simulink model "qnetdcmotor_AhmedMohsin"  (R2022a)
settings: Solver=VariableStepAuto  StartTime=0.0  StopTime=10.0  RelTol=1e-3
InitFcn:
  | R=8.70
  | kt=0.0334
  | ke=0.0334
  | J=1.80e-6
  | L=0.00
  | b=0.00
settings Model: Creator=ahmed  LastModifiedBy=ahmed

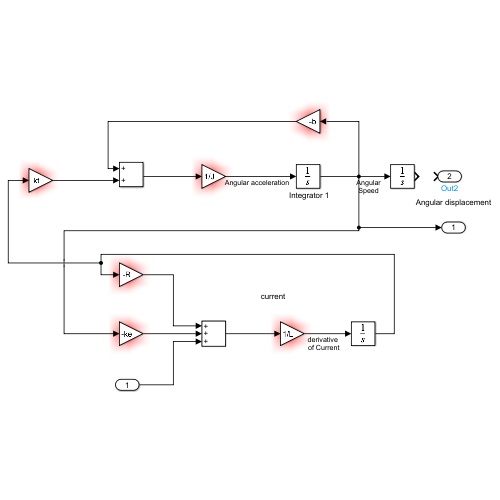
[thumbnail: Simulink's stored preview of the top-level diagram]
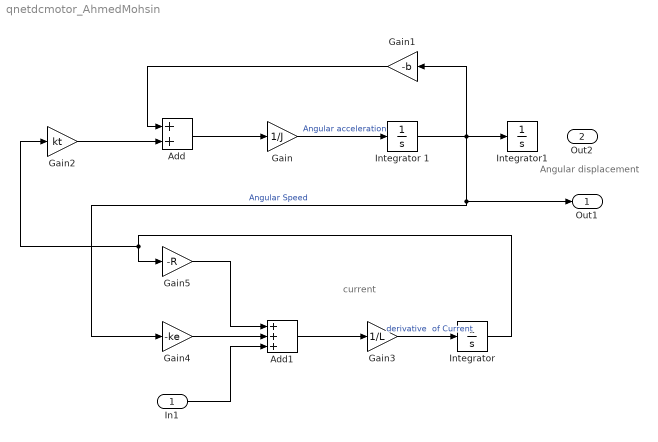
== system qnetdcmotor_AhmedMohsin ==
  note: current
  note: Angular displacement
  In1 : Inport
  " Integrator 1" : Integrator
  Add : Sum
  Add1 : Sum  Inputs=+++
  Gain : Gain  Gain=1/J
  Gain1 : Gain  Gain=-b
  Gain2 : Gain  Gain=kt
  Gain3 : Gain  Gain=1/L
  Gain4 : Gain  Gain=-ke
  Gain5 : Gain  Gain=-R
  Integrator : Integrator
  Integrator1 : Integrator
  Out1 : Outport
  Out2 : Outport  Port=2
  wires:
  " Integrator 1"/1 -> Gain4/1, Out1/1, Gain1/1, Integrator1/1  "Angular Speed"
  Gain/1 -> " Integrator 1"/1  "Angular acceleration"
  Add/1 -> Gain/1
  Gain1/1 -> Add/1
  Gain2/1 -> Add/2
  Gain4/1 -> Add1/2
  Gain5/1 -> Add1/1
  Add1/1 -> Gain3/1
  Gain3/1 -> Integrator/1  "derivative  of Current"
  In1/1 -> Add1/3
  Integrator/1 -> Gain2/1, Gain5/1
